simulink model "PMSM"  (R2023b)
settings: Solver=ode1  StartTime=0.0  StopTime=0.1  FixedStep=1e-7  RelTol=1e-3
libraries: spsIGBTDiodeLib x20, spsSeriesRLCBranchLib x10, simulink x7, spsCurrentMeasurementLib x5, spsVoltageMeasurementLib x3, spsGroundLib x1, spsLinearTransformerLib x1, spsPermanentMagnetSynchronousMachineLib x1, spsThreePhaseProgrammableVoltageSourceLib x1, spsThreePhaseSeriesRLCBranchLib x1, spsThreePhaseVIMeasurementLib x1, spspowerguiLib x1
settings Model: Creator=Marek  LastModifiedBy=Marek

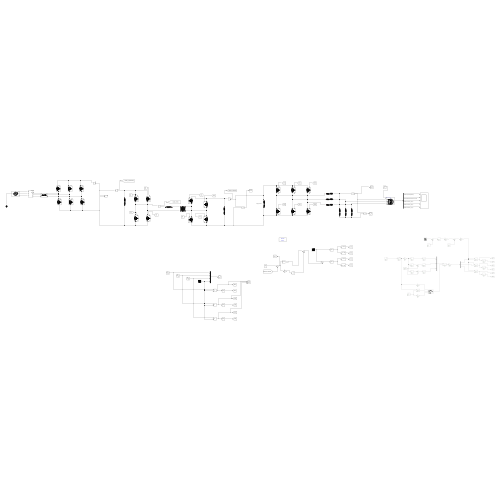
[thumbnail: Simulink's stored preview of the top-level diagram]
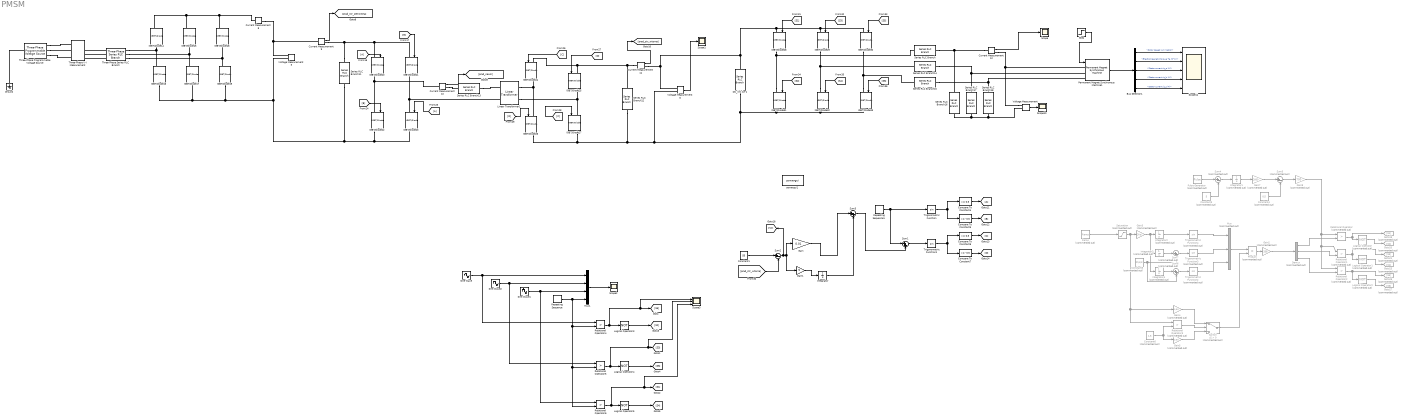
== system PMSM ==
  Bus Selector1 : BusSelector  OutputSignals=Rotor speed wm (rad/s),Electromagnetic torque Te (N*m),Stator current is_a (A),Stator current is_b (A),Stator current is_c (A)
  Compare To Constant4 : simulink/Logic and Bit Operations/Compare To Constant  relop=>=  const=0.5  OutDataTypeStr=boolean
  Compare To Constant5 : simulink/Logic and Bit Operations/Compare To Constant  relop=<=  const=-0.5  OutDataTypeStr=boolean
  Compare To Constant6 : simulink/Logic and Bit Operations/Compare To Constant  relop=>=  const=0.5  OutDataTypeStr=boolean
  Compare To Constant7 : simulink/Logic and Bit Operations/Compare To Constant  relop=<=  const=-0.5  OutDataTypeStr=boolean
  Constant1 : Constant  Value=55
  Constant3 : Constant  Commented=on  Value=5
  Constant4 : Constant  Commented=on  Value=0.5
  Constant5 : Constant  Commented=on  Value=2*pi/3
  Constant6 : Constant  Commented=on  Value=1.5
  Current Measurement{8..12} (5 alike) : spsCurrentMeasurementLib/Current Measurement  PhasorSimulation=off  OutputType=Complex  PSBequivalent=0
  DC_link 1e-1 : spsSeriesRLCBranchLib/Series RLC Branch  LConnTagsString=__new0  RConnTagsString=__new0  BranchType=RC  Resistance=0.01  Inductance=100e-3  SetiL0=off  InitialCurrent=0  Capacitance=1e-3  Setx0=off  InitialVoltage=0  Measurements=None
  Demux : Demux  Commented=on  Outputs=3
  From16 : From
  From25 : From
  Gain : Gain  Gain=0.01
  Gain1 : Gain  Gain=5
  Gain2 : Gain  Commented=on  Gain=338
  Gain3 : Gain  Commented=on  Gain=2*pi
  Gain4 : Gain  Commented=on  Gain=1/50
  Gain5 : Gain  Commented=on  Gain=1/50
  Gain7 : Gain  Commented=on  Gain=2000
  Gain8 : Gain  Commented=on  Gain=700
  Goto11 : Goto
  Goto19 : Goto  Commented=on  GotoTag=S1
  Goto20 : Goto  Commented=on  GotoTag=S2
  Goto21 : Goto  Commented=on  GotoTag=S3
  Goto25 : Goto  Commented=on  GotoTag=S4
  Goto26 : Goto  Commented=on  GotoTag=S5
  Goto27 : Goto  Commented=on  GotoTag=S6
  Ground : spsGroundLib/Ground  LConnTagsString=a
  IGBT/Diode{14..19} (6 alike) : spsIGBTDiodeLib/IGBT//Diode  Ron=1e-3  Rs=1e5  Cs=inf  Measurements=off
  IGBT/Diode{20..33} (14 alike) : spsIGBTDiodeLib/IGBT//Diode  Ron=1e-3  Rs=1e5  Cs=inf  Measurements=on
  Integrator : Integrator
  Integrator{1..4} (4 alike) : Integrator  Commented=on
  Linear Transformer1 : spsLinearTransformerLib/Linear Transformer  UNITS=SI  NominalPower=[ 50e3 5e3 ]  winding1=[400 0 0]  winding2=[290 0 50e-6]  ThreeWindings=off  winding3=[3.15e+05 0.7938 0.084225]  RmLm=[1e6 inf]  Measurements=None  DataType=on
  Logical Operator : Logic  Commented=on  Operator=NOT  AllPortsSameDT=off  OutDataTypeStr=boolean
  Logical Operator1 : Logic  Commented=on  Operator=NOT  Inputs=1  AllPortsSameDT=off  OutDataTypeStr=boolean
  Logical Operator2 : Logic  Commented=on  Operator=NOT  AllPortsSameDT=off  OutDataTypeStr=boolean
  Logical Operator3 : Logic  Operator=NOT  AllPortsSameDT=off  OutDataTypeStr=boolean
  Logical Operator4 : Logic  Operator=NOT  AllPortsSameDT=off  OutDataTypeStr=boolean
  Logical Operator5 : Logic  Operator=NOT  AllPortsSameDT=off  OutDataTypeStr=boolean
  Mux : Mux  Commented=on  Inputs=3
  Mux1 : Mux
  Permanent Magnet Synchronous Machine1 : spsPermanentMagnetSynchronousMachineLib/Permanent Magnet Synchronous Machine  NbPhases=3  FluxDistribution=Sinusoidal  RotorType=Round  MechanicalLoad=Torque Tm  PresetModel="07:  20 Nm 300 Vdc 2200 RPM - 33.9 Nm"  ShowDetailedParameters=on  MeasurementBus=off  Resistance=0.129  Inductance=8.5e-3  dqInductances=[8.5e-3,8.5e-3]  La=0.00153  MachineConstant=Flux linkage established by magnets (V.s)  Flux=0.1821  VoltageCst=132.1171  TorqueCst=1.0926  Flat=120  Mechanical=[0.003334 0.000425 4 0]  PolePairs=4  InitialConditions=[0,0, 0,0]  InitialConditions5ph=[0 0 0 0 0 0]  RefAngle=90 degrees behind phase A axis (modified Park)  IterativeDiscreteModel=Trapezoidal non iterative  TsBlock=-1  TsPowergui=0
  Product : Product  Commented=on
  Pulse Generator : DiscretePulseGenerator  Commented=on  PulseType=Time based  Amplitude=10  Period=2e-4  PulseWidth=50
  Ramp : simulink/Sources/Ramp  Commented=on  slope=50  start=0  InitialOutput=0
  Relational Operator{,1..3} (4 alike) : RelationalOperator  Commented=on  Operator=>  OutDataTypeStr=boolean  RndMeth=Simplest  InputSameDT=off
  Relational Operator4 : RelationalOperator  Operator=>  OutDataTypeStr=boolean  RndMeth=Simplest  InputSameDT=off
  Relational Operator5 : RelationalOperator  Operator=>  OutDataTypeStr=boolean  RndMeth=Simplest  InputSameDT=off
  Relational Operator6 : RelationalOperator  Operator=>  OutDataTypeStr=boolean  RndMeth=Simplest  InputSameDT=off
  Repeating Sequence : simulink/Sources/Repeating Sequence  rep_seq_t=[0 1 2 3]*[1/6000]  rep_seq_y=[0 1 -1 0]
  Repeating Sequence1 : simulink/Sources/Repeating Sequence  rep_seq_t=[0 0.0002]  rep_seq_y=[0 2*pi]
  Saturation : Saturate  Commented=on  UpperLimit=50  LowerLimit=0
  Scope{,1..2,10} (4 alike) : Scope
  Scope11 : Scope  NumInputPorts=5
  Scope3 : Scope  NumInputPorts=3
  Series RLC Branch : spsSeriesRLCBranchLib/Series RLC Branch  LConnTagsString=__new0  RConnTagsString=__new0  BranchType=RL  Resistance=1  Inductance=2.2e-3  SetiL0=off  InitialCurrent=0  Capacitance=1e-6  Setx0=off  InitialVoltage=0  Measurements=None
  Series RLC Branch11 : spsSeriesRLCBranchLib/Series RLC Branch  LConnTagsString=__new0  RConnTagsString=__new0  BranchType=RC  Resistance=0.002  Inductance=1e-3  SetiL0=off  InitialCurrent=0  Capacitance=9e-3  Setx0=on  InitialVoltage=400  Measurements=None
  Series RLC Branch12 : spsSeriesRLCBranchLib/Series RLC Branch  LConnTagsString=__new0  RConnTagsString=__new0  BranchType=RC  Resistance=0.002  Inductance=1e-3  SetiL0=off  InitialCurrent=0  Capacitance=9e-3  Setx0=on  InitialVoltage=290  Measurements=None
  Series RLC Branch13 : spsSeriesRLCBranchLib/Series RLC Branch  LConnTagsString=__new0  RConnTagsString=__new0  BranchType=L  Resistance=0.002  Inductance=100e-6  SetiL0=on  InitialCurrent=30  Capacitance=9e-3  Setx0=on  InitialVoltage=800  Measurements=None
  Series RLC Branch14 : spsSeriesRLCBranchLib/Series RLC Branch  LConnTagsString=__new0  RConnTagsString=__new0  BranchType=RL  Resistance=1  Inductance=2.2e-3  SetiL0=off  InitialCurrent=0  Capacitance=1e-6  Setx0=off  InitialVoltage=0  Measurements=None
  Series RLC Branch15 : spsSeriesRLCBranchLib/Series RLC Branch  LConnTagsString=__new0  RConnTagsString=__new0  BranchType=RL  Resistance=1  Inductance=2.2e-3  SetiL0=off  InitialCurrent=0  Capacitance=1e-6  Setx0=off  InitialVoltage=0  Measurements=None
  Series RLC Branch16 : spsSeriesRLCBranchLib/Series RLC Branch  LConnTagsString=__new0  RConnTagsString=__new0  BranchType=RC  Resistance=1  Inductance=1e-3  SetiL0=off  InitialCurrent=0  Capacitance=10e-6  Setx0=off  InitialVoltage=0  Measurements=None
  Series RLC Branch17 : spsSeriesRLCBranchLib/Series RLC Branch  LConnTagsString=__new0  RConnTagsString=__new0  BranchType=RC  Resistance=1  Inductance=1e-3  SetiL0=off  InitialCurrent=0  Capacitance=10e-6  Setx0=off  InitialVoltage=0  Measurements=None
  Series RLC Branch18 : spsSeriesRLCBranchLib/Series RLC Branch  LConnTagsString=__new0  RConnTagsString=__new0  BranchType=RC  Resistance=1  Inductance=1e-3  SetiL0=off  InitialCurrent=0  Capacitance=10e-6  Setx0=off  InitialVoltage=0  Measurements=None
  Sine Wave : Sin  Frequency=2*pi*50  SampleTime=0
  Sine Wave1 : Sin  Frequency=2*pi*50  Phase=2*pi/3  SampleTime=0
  Sine Wave2 : Sin  Frequency=2*pi*50  Phase=4*pi/3  SampleTime=0
  Step : Step  Time=0.2  Before=1  After=3  SampleTime=0
  Sum1 : Sum  Inputs=|++
  Sum2 : Sum  Inputs=|+-
  Sum3 : Sum  Inputs=|++
  Sum4 : Sum  Commented=on  Inputs=|+-
  Sum5 : Sum  Commented=on  Inputs=|+-
  Sum6 : Sum  Commented=on  Inputs=|++
  Sum7 : Sum  Commented=on  Inputs=|+-
  Switch : Switch  Commented=on  Criteria=u2 > Threshold  ZeroCross=off  SaturateOnIntegerOverflow=off  InputSameDT=off
  Three-Phase Programmable Voltage Source : spsThreePhaseProgrammableVoltageSourceLib/Three-Phase Programmable Voltage Source  PositiveSequence="[400  0 50]"  VariationEntity=None  VariationType=Table of time-amplitude pairs  VariationTypeAlt=Step  VariationStep=0.5  VariationRate=10  VariationMagnitude=0.3  VariationFrequency=2  VariationTiming=[1 2]  VariationPhaseA=off  Amplitudes=[1 0.8 1.2 1.0]  TimeValues=[0 0.1 0.15 0.2]  HarmonicGeneration=off  HarmonicA=[3 0.2 -25 0]  HarmonicB=[2 0.15 35 2]  Timing="[0.05  3]"  BusType=swing  Pref=0  Qref=0  Qmin=-inf  Qmax=inf
  Three-Phase Series RLC Branch : spsThreePhaseSeriesRLCBranchLib/Three-Phase Series RLC Branch  LConnTagsString=A|B|C  RConnTagsString=A|B|C  BranchType=RL  Resistance=1  Inductance=1e-3  Capacitance=1e-6  Measurements=None
  Three-Phase V-I Measurement : spsThreePhaseVIMeasurementLib/Three-Phase V-I Measurement  VoltageMeasurement=phase-to-ground  SetLabelV=off  LabelV=Vabc  Vpu=off  VpuLL=off  CurrentMeasurement=yes  SetLabelI=off  LabelI=Iabc  Ipu=off  Pbase=100e6  Vbase=500e3  OutputType=Complex  PhasorSimulation=off  PSBequivalent=0
  Trigonometric Function : Trigonometry
  Trigonometric Function1 : Trigonometry
  Trigonometric Function2 : Trigonometry  Commented=on
  Trigonometric Function3 : Trigonometry  Commented=on
  Trigonometric Function4 : Trigonometry  Commented=on
  Voltage Measurement : spsVoltageMeasurementLib/Voltage Measurement  PhasorSimulation=off  OutputType=Complex  PSBequivalent=0
  Voltage Measurement5 : spsVoltageMeasurementLib/Voltage Measurement  PhasorSimulation=off  OutputType=Complex  PSBequivalent=0
  Voltage Measurement6 : spsVoltageMeasurementLib/Voltage Measurement  PhasorSimulation=off  OutputType=Complex  PSBequivalent=0
  powergui1 : spspowerguiLib/powergui  Priority=1  SimulationMode=Discrete  SampleTime=1e-6  frequency=60  Iterations=50  frequencyindice=0  Pbase=100e6  ErrMax=1e-4  UnitsV=kV  UnitsW=MW  buscounter=0  FunctionMessages=off  echomessages=off  EnableUseOfTLC=off  CurrentSourceSwitches=off  DisableSnubberDevices=off  DisableRonSwitches=off  DisableVfSwitches=off  DisplayEquations=off  AutomaticDiscreteSolvers=off  SolverType=Tustin/Backward Euler (TBE)  Interpol=off  ExternalGateDelay=off  methode=off  Ts=100  x0status=blocks  SPID=on  SwTol=0  HookPort=off  NonlinearTolerance=1e-4  nMaxIteration=100  ContinueOnMaxIteration=off  RestoreLinks=warning  ResistiveCurrentMeasurement=off  Frange=[0:2:500]  Ylog=off  Xlog=on  ShowGrid=off  save=off  variable=ZData  structure=0  ZoomFFT=off  StartTime=0.0  cycles=1  DisplayStyle=1  fundamental=60  FreqAxis=off  MaxFrequency=1000  frequencyindicesteady=1  RmsSteady=1  display=off
  wires:
  Pulse Generator/1 -> Sum4/1
  Trigonometric Function4/1 -> Mux/1
  Integrator1/1 -> Gain7/1
  Constant4/1 -> Sum5/2
  Constant6/1 -> Gain5/1, Relational Operator3/2
  Gain2/1 -> Demux/1
  Gain8/1 -> Relational Operator/1, Relational Operator1/1, Relational Operator2/1
  Demux/3 -> Relational Operator2/2
  Product/1 -> Gain2/1
  Relational Operator/1 -> Goto19/1, Logical Operator/1
  Sum7/1 -> Trigonometric Function3/1
  Integrator3/1 -> Sum7/1
  Constant5/1 -> Sum6/2, Sum7/2
  Demux/2 -> Relational Operator1/2
  Integrator2/1 -> Trigonometric Function4/1
  Sum6/1 -> Trigonometric Function2/1
  Sum4/1 -> Integrator1/1
  Bus Selector1/5 -> Scope11/5  "<Stator current is_c (A)>"
  Bus Selector1/4 -> Scope11/4  "<Stator current is_b (A)>"
  Bus Selector1/2 -> Scope11/2  "<Electromagnetic torque Te (N*m)>"
  Permanent Magnet Synchronous Machine1/1 -> Bus Selector1/1
  Step/1 -> Permanent Magnet Synchronous Machine1/1
  Bus Selector1/1 -> Scope11/1  "<Rotor speed wm (rad/s)>"
  Bus Selector1/3 -> Scope11/3  "<Stator current is_a (A)>"
  Trigonometric Function/1 -> Compare To Constant5/1, Compare To Constant4/1
  Compare To Constant6/1 -> [C]
  Sum1/1 -> Trigonometric Function1/1
  Compare To Constant4/1 -> Goto11/1
  Trigonometric Function2/1 -> Mux/3
  Sum3/1 -> Sum1/2
  Trigonometric Function1/1 -> Compare To Constant7/1, Compare To Constant6/1
  Compare To Constant5/1 -> [B]
  Gain/1 -> Sum3/1
  Constant1/1 -> Sum2/1
  Sum2/1 -> [nw], Gain1/1, Gain/1
  Relational Operator2/1 -> Goto26/1, Logical Operator2/1
  Compare To Constant7/1 -> [D]
  Gain4/1 -> Switch/1
  Gain7/1 -> Sum5/1
  Switch/1 -> Product/2
  Gain3/1 -> Integrator2/1, Integrator3/1, Integrator4/1
  Logical Operator/1 -> Goto20/1
  Trigonometric Function3/1 -> Mux/2
  Gain5/1 -> Switch/3
  [B] -> IGBT/Diode22/1
  [D] -> IGBT/Diode25/1
  From16/1 -> IGBT/Diode20/1
  [B] -> IGBT/Diode21/1
  [C] -> IGBT/Diode27/1
  From25/1 -> IGBT/Diode23/1
  Current Measurement10/1 -> [prad_cewki]
  Current Measurement11/1 -> [prad_str_wtorna]
  [S5] -> IGBT/Diode30/1
  [S1] -> IGBT/Diode28/1
  [S6] -> IGBT/Diode33/1
  [S4] -> IGBT/Diode32/1
  Current Measurement12/1 -> Scope/1
  Voltage Measurement/1 -> Scope10/1
  [S2] -> IGBT/Diode31/1
  Relational Operator1/1 -> Logical Operator1/1, Goto21/1
  Demux/1 -> Relational Operator/2
  [prad_str_wtorna] -> Sum2/2
  Logical Operator1/1 -> Goto25/1
  [C] -> IGBT/Diode24/1
  [S3] -> IGBT/Diode29/1
  Logical Operator2/1 -> Goto27/1
  Relational Operator3/1 -> Switch/2
  [D] -> IGBT/Diode26/1
  Gain1/1 -> Integrator/1
  Integrator4/1 -> Sum6/1
  Current Measurement9/1 -> [prad_str_pierwotna]
  Constant3/1 -> Sum4/2
  Repeating Sequence1/1 -> Sum1/1, Trigonometric Function/1
  Integrator/1 -> Sum3/2
  Saturation/1 -> Gain4/1, Relational Operator3/1, Gain3/1
  Sum5/1 -> Gain8/1
  Mux/1 -> Product/1
  Ramp/1 -> Saturation/1
  Voltage Measurement6/1 -> Scope1/1
  Relational Operator5/1 -> Scope3/2, [S3], Logical Operator4/1
  Sine Wave/1 -> Relational Operator4/1, Mux1/1
  Sine Wave1/1 -> Mux1/3, Relational Operator6/1
  Mux1/1 -> Scope2/1
  Logical Operator3/1 -> [S2]
  Repeating Sequence/1 -> Mux1/4, Relational Operator6/2, Relational Operator5/2, Relational Operator4/2
  Logical Operator4/1 -> [S6]
  Relational Operator6/1 -> Logical Operator5/1, Scope3/3, [S1]
  Relational Operator4/1 -> Logical Operator3/1, Scope3/1, [S5]
  Logical Operator5/1 -> [S4]
  Sine Wave2/1 -> Mux1/2, Relational Operator5/1
  connections:
  IGBT/Diode27/RConn1 -- IGBT/Diode26/RConn1 -- Series RLC Branch12/RConn1 -- Voltage Measurement6/LConn2 -- DC_link 1e-1/RConn1 -- IGBT/Diode33/RConn1 -- IGBT/Diode32/RConn1 -- IGBT/Diode31/RConn1
  Current Measurement11/RConn1 -- Voltage Measurement6/LConn1 -- DC_link 1e-1/LConn1 -- IGBT/Diode28/LConn1 -- IGBT/Diode30/LConn1 -- IGBT/Diode29/LConn1
  Series RLC Branch17/LConn1 -- Series RLC Branch14/RConn1 -- Permanent Magnet Synchronous Machine1/LConn2
  IGBT/Diode33/LConn1 -- IGBT/Diode30/RConn1 -- Series RLC Branch15/LConn1
  Series RLC Branch18/RConn1 -- Series RLC Branch16/RConn1 -- Series RLC Branch17/RConn1 -- Voltage Measurement/LConn2
  Series RLC Branch11/LConn1 -- Current Measurement9/RConn1 -- IGBT/Diode21/LConn1 -- IGBT/Diode20/LConn1
  Current Measurement11/LConn1 -- IGBT/Diode24/LConn1 -- IGBT/Diode25/LConn1 -- Series RLC Branch12/LConn1
  Voltage Measurement/LConn1 -- Current Measurement12/RConn1 -- Permanent Magnet Synchronous Machine1/LConn1
  IGBT/Diode24/RConn1 -- Linear Transformer1/RConn1 -- IGBT/Diode26/LConn1
  IGBT/Diode20/RConn1 -- Current Measurement10/LConn1 -- IGBT/Diode22/LConn1
  Current Measurement12/LConn1 -- Series RLC Branch/RConn1 -- Series RLC Branch16/LConn1
  IGBT/Diode17/LConn1 -- Three-Phase Series RLC Branch/RConn2 -- IGBT/Diode15/RConn1
  IGBT/Diode21/RConn1 -- IGBT/Diode23/LConn1 -- Linear Transformer1/LConn2
  IGBT/Diode31/LConn1 -- IGBT/Diode28/RConn1 -- Series RLC Branch/LConn1
  Series RLC Branch18/LConn1 -- Permanent Magnet Synchronous Machine1/LConn3 -- Series RLC Branch15/RConn1
  IGBT/Diode14/LConn1 -- IGBT/Diode18/LConn1 -- Current Measurement8/LConn1 -- IGBT/Diode15/LConn1
  IGBT/Diode25/RConn1 -- IGBT/Diode27/LConn1 -- Linear Transformer1/RConn2
  IGBT/Diode14/RConn1 -- Three-Phase Series RLC Branch/RConn1 -- IGBT/Diode16/LConn1
  IGBT/Diode32/LConn1 -- IGBT/Diode29/RConn1 -- Series RLC Branch14/LConn1
  IGBT/Diode16/RConn1 -- IGBT/Diode19/RConn1 -- Voltage Measurement5/LConn2 -- IGBT/Diode22/RConn1 -- IGBT/Diode23/RConn1 -- Series RLC Branch11/RConn1 -- IGBT/Diode17/RConn1
  IGBT/Diode19/LConn1 -- Three-Phase Series RLC Branch/RConn3 -- IGBT/Diode18/RConn1
  Series RLC Branch13/LConn1 -- Linear Transformer1/LConn1
  Ground/LConn1 -- Three-Phase Programmable Voltage Source/LConn1
  Three-Phase Programmable Voltage Source/RConn2 -- Three-Phase V-I Measurement/LConn2
  Current Measurement10/RConn1 -- Series RLC Branch13/RConn1
  Three-Phase Series RLC Branch/LConn2 -- Three-Phase V-I Measurement/RConn2
  Three-Phase Series RLC Branch/LConn3 -- Three-Phase V-I Measurement/RConn3
  Three-Phase Series RLC Branch/LConn1 -- Three-Phase V-I Measurement/RConn1
  Current Measurement8/RConn1 -- Current Measurement9/LConn1 -- Voltage Measurement5/LConn1
  Three-Phase Programmable Voltage Source/RConn1 -- Three-Phase V-I Measurement/LConn1
  Three-Phase Programmable Voltage Source/RConn3 -- Three-Phase V-I Measurement/LConn3
